simulink model "verify_Radiation_Division_mdl"  (R2018b)
settings: Solver=VariableStepAuto  StartTime=0.0  StopTime=365*24*3600  MaxStep=100  RelTol=1e-3  EnableMultiTasking=on
undefined symbols (not defined in the file or in its folder): path_carnot
libraries: carnot x2
settings Model: Creator=drhf  LastModifiedBy=drhf
settings DataIOCC: SaveFormat=Array  SignalLoggingSaveFormat=ModelDataLogs
settings OptimizationCC: ExpressionDepthLimit=2147483647  LifeSpan=inf
settings DebuggingCC: UnderspecifiedInitializationDetection=Classic  MergeDetectMultiDrivingBlocksExec=none  SolverPrmCheckMsg=warning  FcnCallInpInsideContextMsg=warning  StateNameClashWarn=warning  SFUnexpectedBacktrackingDiag=warning  SFNoUnconditionalDefaultTransitionDiag=warning  SFExecutionAtInitializationDiag=none
settings HardwareCC: ProdBitPerPointer=32  ProdBitPerSizeT=32  ProdBitPerPtrDiffT=32  ProdLargestAtomicFloat=None  ProdIntDivRoundTo=Undefined  ProdEndianess=Unspecified  ProdWordSize=32  ProdHWDeviceType=32-bit Generic
settings ModelReferenceCC: PropagateSignalLabelsOutOfModel=off
settings SFSimCC: SimUseLocalCustomCode=off
settings RTWCC: RTWUseLocalCustomCode=off
settings CodeAppCC: StateflowObjectComments=on
settings GRTTargetCC: TargetLangStandard=C89/C90 (ANSI)  GeneratePreprocessorConditionals=Disable all  CombineOutputUpdateFcns=off  GRTInterface=on
settings ConfigComp: CovMetricSettings=dw  CovHtmlReporting=on  CovSaveCumulativeToWorkspaceVar=on  CovSaveSingleToWorkspaceVar=on  CovExternalEMLEnable=off

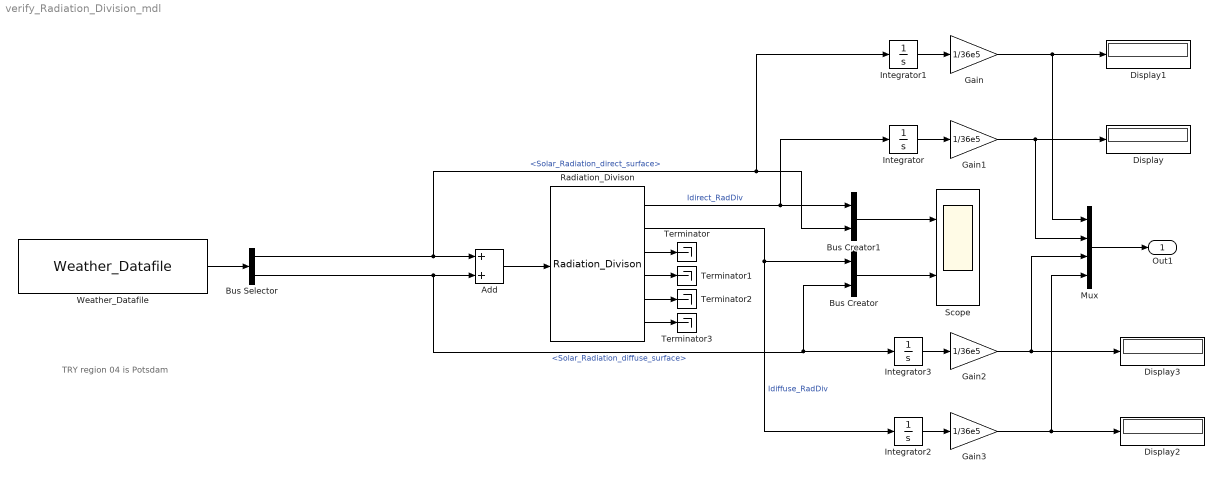
== system verify_Radiation_Division_mdl ==
  note: TRY region 04 is Potsdam
  Add : Sum
  Bus Creator : BusCreator  Inputs=2
  Bus Creator1 : BusCreator  Inputs=2
  Bus Selector : BusSelector  OutputSignals=Solar_Radiation_direct_surface,Solar_Radiation_diffuse_surface
  Display{,1..3} (4 alike) : Display
  Gain{,1..3} (4 alike) : Gain  Gain=1/36e5
  Integrator{,1..3} (4 alike) : Integrator
  Mux : Mux
  Radiation_Divison : carnot/Basic/Weather_and_Sun/Radiation_Divison  latitude=52.383333 % Potsdam  longitude=-13.066667 % Potsdam  longitude0="-15  % CET"
      settings: SourceProductName=Carnot
  Scope : Scope  NumInputPorts=2
  Terminator{,1..3} (4 alike) : Terminator
  Weather_Datafile : carnot/Weather/Weather_Datafile  PathName=path_carnot('data')  FileName='DE_TRY2010_04_averageYear.mat'  UserParam=off  VariableName=DE_TRY2010_04_averageYear  SampleTime=3600
      settings: SourceProductName=Carnot
  Out1 : Outport
  wires:
  Gain/1 -> Mux/1, Display1/1
  Radiation_Divison/3 -> Terminator/1
  Integrator3/1 -> Gain2/1
  Weather_Datafile/1 -> Bus Selector/1
  Add/1 -> Radiation_Divison/1
  Bus Creator/1 -> Scope/2
  Gain2/1 -> Mux/3, Display3/1
  Gain1/1 -> Mux/2, Display/1
  Integrator1/1 -> Gain/1
  Integrator/1 -> Gain1/1
  Integrator2/1 -> Gain3/1
  Bus Selector/2 -> Integrator3/1, Bus Creator/2, Add/2  "<Solar_Radiation_diffuse_surface>"
  Gain3/1 -> Mux/4, Display2/1
  Radiation_Divison/2 -> Integrator2/1, Bus Creator/1  "Idiffuse_RadDiv"
  Bus Selector/1 -> Integrator1/1, Bus Creator1/2, Add/1  "<Solar_Radiation_direct_surface>"
  Radiation_Divison/1 -> Integrator/1, Bus Creator1/1  "Idirect_RadDiv"
  Bus Creator1/1 -> Scope/1
  Radiation_Divison/5 -> Terminator2/1
  Radiation_Divison/4 -> Terminator1/1
  Mux/1 -> Out1/1
  Radiation_Divison/6 -> Terminator3/1
